simulink library "mbd_s32k1xx_ec_toolbox"  (Simulink 9.0)
settings: Solver=FixedStepDiscrete  StartTime=0.0  StopTime=10.0  FixedStep=0.1  RelTol=1e-3  EnableMultiTasking=on
InitFcn:
  | mbd_s32k_consistency_checks(bdroot(gcs));
(part 1 of 8)
settings Model: Creator=r61406  LastModifiedBy=nxf35172

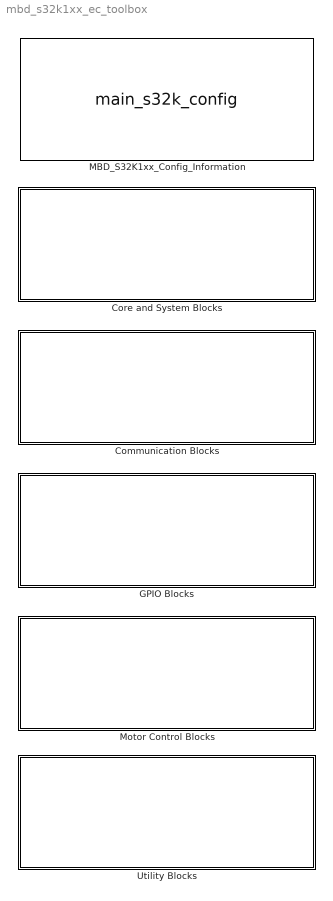
== system mbd_s32k1xx_ec_toolbox ==
  Communication Blocks : Subsystem
  Core and System Blocks : Subsystem
  GPIO Blocks : Subsystem
  MBD_S32K1xx_Config_Information : S-Function  LoadFcn=|  InitFcn=|  FunctionName=main_s32k_config  SFunctionDeploymentMode=off  EnableBusSupport=off  mask(MBDTBX_EC_S32K){mbdt_ver=0, disp_str=|, config_params=[], mcu_target_name=S32K148, mcu_target_package=100-LQFP, mcu_target_sram_size=192KB, mcu_system_clock_freq=80, mcu_xtal_freq=External 8, mcu_steptick_timer=LPIT Channel 0, mcu_steptick_prio=15, ds_import_enable=on, target_compiler=GCC, target_memory=FLASH, gcc_target_compile_opts=-mthumb -mfloat-abi=hard -mfpu=fpv4-sp-d16 -O1 -g -gstrict-dwarf, gcc_target_assemble_opts=-mthumb -mfloat-abi=hard -mfpu=fpv4-sp-d16 -g, gcc_target_link_opts=-mthumb -mfloat-abi=hard -mfpu=fpv4-sp-d16, gcc_target_lib_opts=, gcc_target_default_lcf=on, gcc_target_user_lcf=S32K148_192_flash.ld, ghs_target_compile_opts=-cpu=cortexm4f -thumb -fpu=vfpv4_d16 -fsingle -Ogeneral -Wundef -Wimplicit-int -Wshadow -Wtrigraphs --no_commons --gnu_asm -gnu99 -gdwarf-2 -G, ghs_target_assemble_opts=-cpu=cortexm4f -fpu=vfpv4_d16, ghs_target_link_opts=-cpu=cortexm4f -thumb -fpu=vfpv4_d16, ghs_target_lib_opts=, ghs_target_default_lcf=on, ghs_target_user_lcf=S32K148_192_flash.ld, iar_target_compile_opts=--cpu=Cortex-M4F --thumb --fpu=VFPv4_sp -Ol -e --debug --dlib_config normal, iar_target_assemble_opts=--cpu Cortex-M4F --thumb --fpu VFPv4_sp, iar_target_link_opts=--no_exceptions --vfe --inline, iar_target_lib_opts=, iar_target_default_lcf=on, iar_target_user_lcf=S32K148_192_flash.icf, pil_download_enable=off, rbl_download_enable=off, rbl_start_delay=5000, rbl_download_interface=OpenSDA, rbl_restart_request=off, rbl_com_port=Custom, rbl_com_port_custom=COM1, pil_download_rate=57600, pil_opensda_drive=Custom, pil_opensda_drive_custom=D, pil_uart_instance=1, pil_uart_rx=PTC6: [LPUART1_RX | Receive], pil_uart_tx=PTC7: [LPUART1_TX | Transmit], FTM_PWM_PcrCheckEnDis=on, FTM_Input_Edge_Inputs_PcrCheckEnDis=on, FTM_Dual_Edge_Inputs_PcrCheckEnDis=on, FTM_Quadrature_Inputs_PcrCheckEnDis=on, FTM_Hall_Sensor_Inputs_PcrCheckEnDis=on, LPTMR_PcrCheckEnDis=on, PIT_PcrCheckEnDis=on, RTC_PcrCheckEnDis=on, FlexCAN_PcrCheckEnDis=on, LIN_PcrCheckEnDis=on, FlexIO_PcrCheckEnDis=on, LPI2C_PcrCheckEnDis=on, LPSPI_PcrCheckEnDis=on, LPUART_PcrCheckEnDis=on, CMP_PcrCheckEnDis=on, GPIO_OutputPcrCheckEnDis=on, GPIO_InputPcrCheckEnDis=on, SBC_PcrCheckEnDis=on, AMMCLIB_PcrCheckEnDis=on, FM_PcrCheckEnDis=on, Profile_PcrCheckEnDis=on, ConfigParams_PcrCheckEnDis=on, ModelRef_PcrCheckEnDis=on, PDB0_PcrCheckEnDis=on, CSEc_PcrCheckEnDis=on, eDMA_PcrCheckEnDis=on, ADC_PcrCheckEnDis=on, WDOG_PcrCheckEnDis=on}
      LoadFcn=|
      | mbd_s32k_set_cur_model(bdroot(gcs));
      | mbd_s32k_block_load(bdroot(gcs));
      InitFcn=|
      | mbd_s32k_set_cur_model(bdroot(gcs)); 
      | mbd_s32k_update_model('init');       
      | mbd_s32k_check('MBDTBX_EC_S32K14');
      mask disp_str=|
      | Target : S32K144-64KB_SRAM
      | Package : 100-pin
      | System clock : 80 MHz
      | XTAL clock : External 8 MHz
      | Compiler : IAR
      | Target Type : FLASH
      | Download Code after build : off
      | Step Tick Interrupt Priority : 15
      mask prompts: mbdt_ver "MBDT Version"; disp_str "display_string"; mcu_target_name "Family"; mcu_target_package "Package"; mcu_target_sram_size "SRAM"; mcu_system_clock_freq "Clock Frequency MHz"; mcu_xtal_freq "XTAL Frequency MHz"; mcu_steptick_timer "Timer"; mcu_steptick_prio "Priority"; ds_import_enable "Generate S32 Design Studio ProjectInfo.xml file"; target_compiler "Compiler"; target_memory "Target Memory Model"; gcc_target_compile_opts "Compile Options"; gcc_target_assemble_opts "Assemble Options"; gcc_target_link_opts "Link Options"; gcc_target_lib_opts "Library Options"; gcc_target_default_lcf "Default Target Memory Definitions"; gcc_target_user_lcf "User Defined Target Memory Definitions"; ghs_target_compile_opts "Compile Options"; ghs_target_assemble_opts "Assemble Options"; ghs_target_link_opts "Link Options"; ghs_target_lib_opts "Library Options"; ghs_target_default_lcf "Default Target Memory Definitions"; ghs_target_user_lcf "User Defined Target Memory Definitions"; iar_target_compile_opts "Compile Options"; iar_target_assemble_opts "Assemble Options"; iar_target_link_opts "Link Options"; iar_target_lib_opts "Library Options"; iar_target_default_lcf "Default Target Memory Definitions"; iar_target_user_lcf "User Defined Target Memory Definitions"; pil_download_enable "Processor-in-the-Loop (PIL) Mode Download"; rbl_download_enable "Download Code after Build"; rbl_start_delay "Delay before start of application (ms)"; rbl_download_interface "Download Interface"; rbl_restart_request "Boot Assist Module (BAM) Restart Request"; rbl_com_port "COM Port"; rbl_com_port_custom "Custom COM Port"; pil_download_rate "Baud Rate"; pil_opensda_drive "OpenSDA Drive Name"; pil_opensda_drive_custom "Custom OpenSDA Drive Name"; pil_uart_instance "LPUART"; pil_uart_rx "RX pin"; pil_uart_tx "TX pin"; FTM_PWM_PcrCheckEnDis "FTM PWM Config"; FTM_Input_Edge_Inputs_PcrCheckEnDis "FTM Input Edge Inputs"; FTM_Dual_Edge_Inputs_PcrCheckEnDis "FTM Dual Edge Inputs"; FTM_Quadrature_Inputs_PcrCheckEnDis "FTM Quadrature Inputs"; FTM_Hall_Sensor_Inputs_PcrCheckEnDis "FTM Hall Sensor Inputs"; LPTMR_PcrCheckEnDis "LPTMR"; PIT_PcrCheckEnDis "PIT"; RTC_PcrCheckEnDis "RTC"; FlexCAN_PcrCheckEnDis "FlexCAN"; LIN_PcrCheckEnDis "LIN"; FlexIO_PcrCheckEnDis "FlexIO"; LPI2C_PcrCheckEnDis "LPI2C"; LPSPI_PcrCheckEnDis "LPSPI"; LPUART_PcrCheckEnDis "LPUART"; CMP_PcrCheckEnDis "CMP"; GPIO_OutputPcrCheckEnDis "GPIO Output"; GPIO_InputPcrCheckEnDis "GPIO Input"; SBC_PcrCheckEnDis "SBC"; AMMCLIB_PcrCheckEnDis "AMMCLIB"; FM_PcrCheckEnDis "FreeMaster"; Profile_PcrCheckEnDis "Profile"; ConfigParams_PcrCheckEnDis "Config Params"; ModelRef_PcrCheckEnDis "Model Reference"; PDB0_PcrCheckEnDis "PDB"; CSEc_PcrCheckEnDis "CSEc"; eDMA_PcrCheckEnDis "eDMA"; ADC_PcrCheckEnDis "ADC"; WDOG_PcrCheckEnDis "WDOG"
      mask help: Model-Based Design Toolbox Config block for S32K1xx family of processors.
      mask init:
      | mbd_s32k_config_com_ports_cbk('populate_drop_down');
      | maskStr = mbd_s32k_mb_display_string();
      settings: NameChangeFcn=mbd_s32k_model_close;
      settings: CopyFcn=|
      | mbd_s32k_set_cur_model(bdroot(gcs));
      | mbd_s32k_check('MBDTBX_EC_S32K');
      | mbd_s32k_update_model('copy');
      settings: ModelCloseFcn=|
      | mbd_s32k_set_cur_model(bdroot(gcs));
      | mbd_s32k_model_close;
      settings: CloseFcn=|
      | mbd_s32k_set_cur_model(bdroot(gcs));
      | mbd_s32k_check('MBDTBX_EC_S32K');
      | mbd_s32k_update_model('copy');
      mask Help: web(fullfile(mbd_s32k_block_help, 'main_config', 'main_config.html'));
      mask TypeOptions mcu_target_name: S32K116 | S32K118 | S32K142 | S32K144 | S32K146 | S32K148
      mask Callback mcu_target_name:
      | mbd_s32k_config_target_cbk('mcu_target_name');
      | mbd_s32k_config_target_cbk('mcu_target_compiler');
      | mbd_s32k_config_target_cbk('mcu_target_memory');
      mask TypeOptions mcu_target_package: 100-LQFP | 144-LQFP | 176-LQFP | 100-BGA
      mask Callback mcu_target_package: mbd_s32k_config_target_cbk('mcu_target_package')
      mask TypeOptions mcu_target_sram_size: 192KB | 256KB
      mask Callback mcu_target_sram_size: mbd_s32k_config_target_cbk('mcu_target_sram_size')
      mask TypeOptions mcu_system_clock_freq: 80 | 112
      mask TypeOptions mcu_xtal_freq: External 8 | External 40
      mask TypeOptions mcu_steptick_timer: LPIT Channel 0 | Suppress
      mask TypeOptions mcu_steptick_prio: 15 | 14 | 13 | 12 | 11 | 10 | 9 | 8 | 7 | 6 | 5 | 4 | 3 | 2 | 1 | 0
      mask TypeOptions target_compiler: GCC | IAR | GreenHills Multi
      mask Callback target_compiler: mbd_s32k_config_compiler_cbk('target_compiler')
      mask TypeOptions target_memory: FLASH | SRAM
      mask Callback target_memory: mbd_s32k_config_memory_cbk('target_memory')
      mask Callback gcc_target_default_lcf: mbd_s32k_config_lcf_cbk('gcc_target_default_lcf')
      mask TypeOptions gcc_target_user_lcf: S32K148_192_flash.ld | S32K148_192_flash_bam.ld
      mask TypeOptions ghs_target_user_lcf: S32K148_192_flash.ld | S32K148_192_flash_bam.ld
      mask Callback iar_target_default_lcf: mbd_s32k_config_lcf_cbk('iar_target_default_lcf')
      mask TypeOptions iar_target_user_lcf: S32K148_192_flash.icf | S32K148_192_flash_bam.icf
      mask Callback pil_download_enable: mbd_s32k_config_pil_cbk('pil_download_enable')
      mask Callback rbl_download_enable: mbd_s32k_config_pil_cbk('rbl_download_enable');
      mask TypeOptions rbl_download_interface: Serial | OpenSDA
      mask Callback rbl_download_interface: mbd_s32k_config_pil_cbk('rbl_download_interface')
      mask TypeOptions rbl_com_port: COM1 | COM17 | Custom
      mask Callback rbl_com_port: mbd_s32k_config_com_ports_cbk('populate_drop_down')
      mask TypeOptions pil_download_rate: 9600 | 14400 | 19200 | 38400 | 56000 | 57600 | 115200
      mask TypeOptions pil_opensda_drive: D: S32K116EVB | Custom
      mask Callback pil_opensda_drive:
      | mbd_s32k_config_vol_disks_cbk('populate_drop_down');
      | mbd_s32k_config_vol_disks_cbk('enable_custom');
      mask TypeOptions pil_uart_instance: 0 | 1 | 2
      mask Callback pil_uart_instance: mbd_s32k_config_pil_cbk('pil_uart_instance');
      mask TypeOptions pil_uart_rx: PTA2: [LPUART0_RX | Receive] | PTB0: [LPUART0_RX | Receive] | PTC2: [LPUART0_RX | Receive] | PTC6: [LPUART1_RX | Receive] | PTC8: [LPUART1_RX | Receive] | PTA2: [LPUART0_RX | Receive] | PTB0: [LPUART0_RX | Receive] | PTC2: [LPUART0_RX | Receive] | PTC6: [LPUART1_RX | Receive] | PTC8: [LPUART1_RX | Receive] | PTA2: [LPUART0_RX | Receive] | PTB0: [LPUART0_RX | Receive] | PTC2: [LPUART0_RX | Receive] | PTC6: [LPUART1_RX | Receive] | PTC8: [LPUART1_RX | Receive] | PTA2: [LPUART0_RX | Receive] | PTB0: [LPUART0_RX | Receive] | PTC2: [LPUART0_RX | Receive] | PTC6: [LPUART1_RX | Receive] | PTC8: [LPUART1_RX | Receive] | PTA8: [LPUART2_RX | Receive] | PTD6: [LPUART2_RX | Receive] | PTD17: [LPUART2_RX | Receive] | PTA2: [LPUART0_RX | Receive] | PTB0: [LPUART0_RX | Receive] | PTC2: [LPUART0_RX | Receive] | PTC6: [LPUART1_RX | Receive] | PTC8: [LPUART1_RX | Receive] | PTA8: [LPUART2_RX | Receive] | PTD6: [LPUART2_RX | Receive] | PTD17: [LPUART2_RX | Receive] | PTA2: [LPUART0_RX | Receive] | PTB0: [LPUART0_RX | Receive] | PTC2: [LPUART0_RX | Receive] | PTC6: [LPUART1_RX | Receive] | PTC8: [LPUART1_RX | Receive] | PTA8: [LPUART2_RX | Receive] | PTD6: [LPUART2_RX | Receive] | PTD17: [LPUART2_RX | Receive]
      mask TypeOptions pil_uart_tx: PTA3: [LPUART0_TX | Transmit] | PTB1: [LPUART0_TX | Transmit] | PTC3: [LPUART0_TX | Transmit] | PTC7: [LPUART1_TX | Transmit] | PTC9: [LPUART1_TX | Transmit] | PTA3: [LPUART0_TX | Transmit] | PTB1: [LPUART0_TX | Transmit] | PTC3: [LPUART0_TX | Transmit] | PTC7: [LPUART1_TX | Transmit] | PTC9: [LPUART1_TX | Transmit] | PTA3: [LPUART0_TX | Transmit] | PTB1: [LPUART0_TX | Transmit] | PTC3: [LPUART0_TX | Transmit] | PTC7: [LPUART1_TX | Transmit] | PTC9: [LPUART1_TX | Transmit] | PTA3: [LPUART0_TX | Transmit] | PTB1: [LPUART0_TX | Transmit] | PTC3: [LPUART0_TX | Transmit] | PTC7: [LPUART1_TX | Transmit] | PTC9: [LPUART1_TX | Transmit] | PTA9: [LPUART2_TX | Transmit] | PTD7: [LPUART2_TX | Transmit] | PTE12: [LPUART2_TX | Transmit] | PTA3: [LPUART0_TX | Transmit] | PTB1: [LPUART0_TX | Transmit] | PTC3: [LPUART0_TX | Transmit] | PTC7: [LPUART1_TX | Transmit] | PTC9: [LPUART1_TX | Transmit] | PTA9: [LPUART2_TX | Transmit] | PTD7: [LPUART2_TX | Transmit] | PTE12: [LPUART2_TX | Transmit] | PTA3: [LPUART0_TX | Transmit] | PTB1: [LPUART0_TX | Transmit] | PTC3: [LPUART0_TX | Transmit] | PTC7: [LPUART1_TX | Transmit] | PTC9: [LPUART1_TX | Transmit] | PTA9: [LPUART2_TX | Transmit] | PTD7: [LPUART2_TX | Transmit] | PTE12: [LPUART2_TX | Transmit]
      mask DialogControl Container14 Prompt: Target MCU
      mask DialogControl Container15 Prompt: Clock
      mask DialogControl Container16 Prompt: Step Tick
      mask DialogControl propagate_configuration Prompt: Propagate configuration
      mask DialogControl propagate_configuration Tooltip: Press this button to propagate the settings to all referenced models.
      mask DialogControl propagate_configuration Callback: mbd_s32k_config_propagate_cbk(gcb);
      mask DialogControl rbl_com_button Prompt: Refresh
      mask DialogControl rbl_com_button Callback: mbd_s32k_config_com_ports_cbk('populate_drop_down')
      mask DialogControl pil_opensda_refresh Prompt: Refresh
      mask DialogControl pil_opensda_refresh Callback: mbd_s32k_config_vol_disks_cbk('populate_drop_down')
      mask DialogControl Container17 Prompt: Consistency checks
      mask Display:
      | image('nxp_logo.png', 'top-right');
      | disp(maskStr);
  Motor Control Blocks : Subsystem
  Utility Blocks : Subsystem

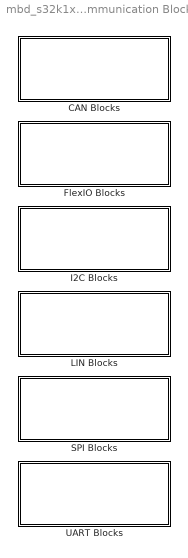
== system mbd_s32k1xx_ec_toolbox/Communication Blocks ==
  CAN Blocks : Subsystem
  "FlexIO Blocks " : Subsystem
  I2C Blocks : Subsystem
  LIN Blocks : Subsystem
  SPI Blocks : Subsystem
  UART Blocks : Subsystem

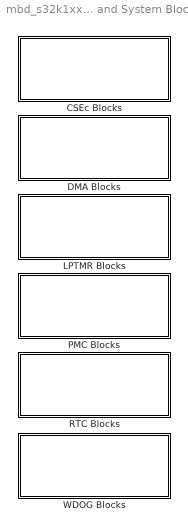
== system mbd_s32k1xx_ec_toolbox/Core and System Blocks ==
  CSEc Blocks : Subsystem
  DMA Blocks : Subsystem
  LPTMR Blocks : Subsystem
  PMC Blocks : Subsystem
  RTC Blocks : Subsystem
  WDOG Blocks : Subsystem

== system mbd_s32k1xx_ec_toolbox/GPIO Blocks ==
  Digital_Input : S-Function  FunctionName=gpio_s32k_input  SFunctionDeploymentMode=off  EnableBusSupport=off  mask(gpio_s32k_input){gpio_pin=PTA0: [PTA0 | Port A I/O], pull_resistor=None, passive_filter=off}
      mask prompts: gpio_pin "Input Pin"; pull_resistor "Pull Resistor Select"; passive_filter "Passive Filter Enable"
      mask help: Select a General Purpose Input Pin as a Source.
      mask init:
      | mbd_s32k_gpi_init;
      settings: NameChangeFcn=mbd_s32k_name_check (gcb);
      mask Help: web(fullfile(mbd_s32k_block_help, 'gpio', 'gpio_input.html'));
      mask TypeOptions gpio_pin: PTA0: [PTA0 | Port A I/O] | PTA1: [PTA1 | Port A I/O] | PTA2: [PTA2 | Port A I/O] | PTA3: [PTA3 | Port A I/O] | PTA4: [PTA4 | Port A I/O] | PTA5: [PTA5 | Port A I/O] | PTA6: [PTA6 | Port A I/O] | PTA7: [PTA7 | Port A I/O] | PTA8: [PTA8 | Port A I/O] | PTA9: [PTA9 | Port A I/O] | PTA10: [PTA10 | Port A I/O] | PTA11: [PTA11 | Port A I/O] | PTA12: [PTA12 | Port A I/O] | PTA13: [PTA13 | Port A I/O] | PTA14: [PTA14 | Port A I/O] | PTA15: [PTA15 | Port A I/O] | PTA16: [PTA16 | Port A I/O] | PTA17: [PTA17 | Port A I/O] | PTA18: [PTA18 | Port A I/O] | PTA19: [PTA19 | Port A I/O] | PTA20: [PTA20 | Port A I/O] | PTA21: [PTA21 | Port A I/O] | PTA22: [PTA22 | Port A I/O] | PTA23: [PTA23 | Port A I/O] | PTA24: [PTA24 | Port A I/O] | PTA25: [PTA25 | Port A I/O] | PTA26: [PTA26 | Port A I/O] | PTA27: [PTA27 | Port A I/O] | PTA28: [PTA28 | Port A I/O] | PTA29: [PTA29 | Port A I/O] | PTA30: [PTA30 | Port A I/O] | PTA31: [PTA31 | Port A I/O] | PTB0: [PTB0 | Port B I/O] | PTB1: [PTB1 | Port B I/O] | PTB2: [PTB2 | Port B I/O] | PTB3: [PTB3 | Port B I/O] | PTB4: [PTB4 | Port B I/O] | PTB5: [PTB5 | Port B I/O] | PTB6: [PTB6 | Port B I/O] | PTB7: [PTB7 | Port B I/O] | PTB8: [PTB8 | Port B I/O] | PTB9: [PTB9 | Port B I/O] | PTB10: [PTB10 | Port B I/O] | PTB11: [PTB11 | Port B I/O] | PTB12: [PTB12 | Port B I/O] | PTB13: [PTB13 | Port B I/O] | PTB14: [PTB14 | Port B I/O] | PTB15: [PTB15 | Port B I/O] | PTB16: [PTB16 | Port B I/O] | PTB17: [PTB17 | Port B I/O] | PTB18: [PTB18 | Port B I/O] | PTB19: [PTB19 | Port B I/O] | PTB20: [PTB20 | Port B I/O] | PTB21: [PTB21 | Port B I/O] | PTB22: [PTB22 | Port B I/O] | PTB23: [PTB23 | Port B I/O] | PTB24: [PTB24 | Port B I/O] | PTB25: [PTB25 | Port B I/O] | PTB26: [PTB26 | Port B I/O] | PTB27: [PTB27 | Port B I/O] | PTB28: [PTB28 | Port B I/O] | PTB29: [PTB29 | Port B I/O] | PTB30: [PTB30 | Port B I/O] | PTB31: [PTB31 | Port B I/O] | PTC0: [PTC0 | Port C I/O] | PTC1: [PTC1 | Port C I/O] | PTC2: [PTC2 | Port C I/O] | PTC3: [PTC3 | Port C I/O] | PTC4: [PTC4 | Port C I/O] | PTC5: [PTC5 | Port C I/O] | PTC6: [PTC6 | Port C I/O] | PTC7: [PTC7 | Port C I/O] | PTC8: [PTC8 | Port C I/O] | PTC9: [PTC9 | Port C I/O] | PTC10: [PTC10 | Port C I/O] | PTC11: [PTC11 | Port C I/O] | PTC12: [PTC12 | Port C I/O] | PTC13: [PTC13 | Port C I/O] | PTC14: [PTC14 | Port C I/O] | PTC15: [PTC15 | Port C I/O] | PTC16: [PTC16 | Port C I/O] | PTC17: [PTC17 | Port C I/O] | PTC18: [PTC18 | Port C I/O] | PTC19: [PTC19 | Port C I/O] | PTC20: [PTC20 | Port C I/O] | PTC21: [PTC21 | Port C I/O] | PTC22: [PTC22 | Port C I/O] | PTC23: [PTC23 | Port C I/O] | PTC24: [PTC24 | Port C I/O] | PTC25: [PTC25 | Port C I/O] | PTC26: [PTC26 | Port C I/O] | PTC27: [PTC27 | Port C I/O] | PTC28: [PTC28 | Port C I/O] | PTC29: [PTC29 | Port C I/O] | PTC30: [PTC30 | Port C I/O] | PTC31: [PTC31 | Port C I/O] | PTD0: [PTD0 | Port D I/O] | PTD1: [PTD1 | Port D I/O] | PTD2: [PTD2 | Port D I/O] | PTD3: [PTD3 | Port D I/O] | PTD4: [PTD4 | Port D I/O] | PTD5: [PTD5 | Port D I/O] | PTD6: [PTD6 | Port D I/O] | PTD7: [PTD7 | Port D I/O] | PTD8: [PTD8 | Port D I/O] | PTD9: [PTD9 | Port D I/O] | PTD10: [PTD10 | Port D I/O] | PTD11: [PTD11 | Port D I/O] | PTD12: [PTD12 | Port D I/O] | PTD13: [PTD13 | Port D I/O] | PTD14: [PTD14 | Port D I/O] | PTD15: [PTD15 | Port D I/O] | PTD16: [PTD16 | Port D I/O] | PTD17: [PTD17 | Port D I/O] | PTD18: [PTD18 | Port D I/O] | PTD19: [PTD19 | Port D I/O] | PTD20: [PTD20 | Port D I/O] | PTD21: [PTD21 | Port D I/O] | PTD22: [PTD22 | Port D I/O] | PTD23: [PTD23 | Port D I/O] | PTD24: [PTD24 | Port D I/O] | PTD25: [PTD25 | Port D I/O] | PTD26: [PTD26 | Port D I/O] | PTD27: [PTD27 | Port D I/O] | PTD28: [PTD28 | Port D I/O] | PTD29: [PTD29 | Port D I/O] | PTD30: [PTD30 | Port D I/O] | PTD31: [PTD31 | Port D I/O] | PTE0: [PTE0 | Port E I/O] | PTE1: [PTE1 | Port E I/O] | PTE2: [PTE2 | Port E I/O] | PTE3: [PTE3 | Port E I/O] | PTE4: [PTE4 | Port E I/O] | PTE5: [PTE5 | Port E I/O] | PTE6: [PTE6 | Port E I/O] | PTE7: [PTE7 | Port E I/O] | PTE8: [PTE8 | Port E I/O] | PTE9: [PTE9 | Port E I/O] | PTE10: [PTE10 | Port E I/O] | PTE11: [PTE11 | Port E I/O] | PTE12: [PTE12 | Port E I/O] | PTE13: [PTE13 | Port E I/O] | PTE14: [PTE14 | Port E I/O] | PTE15: [PTE15 | Port E I/O] | PTE16: [PTE16 | Port E I/O] | PTE17: [PTE17 | Port E I/O] | PTE18: [PTE18 | Port E I/O] | PTE19: [PTE19 | Port E I/O] | PTE20: [PTE20 | Port E I/O] | PTE21: [PTE21 | Port E I/O] | PTE22: [PTE22 | Port E I/O] | PTE23: [PTE23 | Port E I/O] | PTE24: [PTE24 | Port E I/O] | PTE25: [PTE25 | Port E I/O] | PTE26: [PTE26 | Port E I/O] | PTE27: [PTE27 | Port E I/O]
      mask Callback gpio_pin: mbd_s32k_display_pin_info('gpio', gcb, 'gpio_pin')
      mask TypeOptions pull_resistor: None | Pulldown | Pullup
      mask Display:
      | image('nxp_logo.png', 'top-right');
      | port_label('output',1,'input');
      | disp(maskStr);
  Digital_Input_ISR : S-Function  FunctionName=gpi_s32k_isr  SFunctionDeploymentMode=off  EnableBusSupport=off  mask(gpi_s32k_isr){gpio_pin=PTA0: [PTA0 | Port A I/O], irqc=when logic 0, prio=15}
      mask prompts: gpio_pin "Input Pin"; irqc "Interrupt Configuration"; prio "ISR Priority"
      mask help: Configure a General Purpose Input Pin to generate an ISR.
      mask init:
      | mbd_s32k_gpi_isr_init;
      settings: NameChangeFcn=mbd_s32k_name_check (gcb);
      mask Help: web(fullfile(mbd_s32k_block_help, 'gpio', 'gpi_isr.html'));
      mask TypeOptions gpio_pin: PTA0: [PTA0 | Port A I/O] | PTA1: [PTA1 | Port A I/O] | PTA2: [PTA2 | Port A I/O] | PTA3: [PTA3 | Port A I/O] | PTA4: [PTA4 | Port A I/O] | PTA5: [PTA5 | Port A I/O] | PTA6: [PTA6 | Port A I/O] | PTA7: [PTA7 | Port A I/O] | PTA8: [PTA8 | Port A I/O] | PTA9: [PTA9 | Port A I/O] | PTA10: [PTA10 | Port A I/O] | PTA11: [PTA11 | Port A I/O] | PTA12: [PTA12 | Port A I/O] | PTA13: [PTA13 | Port A I/O] | PTA14: [PTA14 | Port A I/O] | PTA15: [PTA15 | Port A I/O] | PTA16: [PTA16 | Port A I/O] | PTA17: [PTA17 | Port A I/O] | PTA18: [PTA18 | Port A I/O] | PTA19: [PTA19 | Port A I/O] | PTA20: [PTA20 | Port A I/O] | PTA21: [PTA21 | Port A I/O] | PTA22: [PTA22 | Port A I/O] | PTA23: [PTA23 | Port A I/O] | PTA24: [PTA24 | Port A I/O] | PTA25: [PTA25 | Port A I/O] | PTA26: [PTA26 | Port A I/O] | PTA27: [PTA27 | Port A I/O] | PTA28: [PTA28 | Port A I/O] | PTA29: [PTA29 | Port A I/O] | PTA30: [PTA30 | Port A I/O] | PTA31: [PTA31 | Port A I/O] | PTB0: [PTB0 | Port B I/O] | PTB1: [PTB1 | Port B I/O] | PTB2: [PTB2 | Port B I/O] | PTB3: [PTB3 | Port B I/O] | PTB4: [PTB4 | Port B I/O] | PTB5: [PTB5 | Port B I/O] | PTB6: [PTB6 | Port B I/O] | PTB7: [PTB7 | Port B I/O] | PTB8: [PTB8 | Port B I/O] | PTB9: [PTB9 | Port B I/O] | PTB10: [PTB10 | Port B I/O] | PTB11: [PTB11 | Port B I/O] | PTB12: [PTB12 | Port B I/O] | PTB13: [PTB13 | Port B I/O] | PTB14: [PTB14 | Port B I/O] | PTB15: [PTB15 | Port B I/O] | PTB16: [PTB16 | Port B I/O] | PTB17: [PTB17 | Port B I/O] | PTB18: [PTB18 | Port B I/O] | PTB19: [PTB19 | Port B I/O] | PTB20: [PTB20 | Port B I/O] | PTB21: [PTB21 | Port B I/O] | PTB22: [PTB22 | Port B I/O] | PTB23: [PTB23 | Port B I/O] | PTB24: [PTB24 | Port B I/O] | PTB25: [PTB25 | Port B I/O] | PTB26: [PTB26 | Port B I/O] | PTB27: [PTB27 | Port B I/O] | PTB28: [PTB28 | Port B I/O] | PTB29: [PTB29 | Port B I/O] | PTB30: [PTB30 | Port B I/O] | PTB31: [PTB31 | Port B I/O] | PTC0: [PTC0 | Port C I/O] | PTC1: [PTC1 | Port C I/O] | PTC2: [PTC2 | Port C I/O] | PTC3: [PTC3 | Port C I/O] | PTC4: [PTC4 | Port C I/O] | PTC5: [PTC5 | Port C I/O] | PTC6: [PTC6 | Port C I/O] | PTC7: [PTC7 | Port C I/O] | PTC8: [PTC8 | Port C I/O] | PTC9: [PTC9 | Port C I/O] | PTC10: [PTC10 | Port C I/O] | PTC11: [PTC11 | Port C I/O] | PTC12: [PTC12 | Port C I/O] | PTC13: [PTC13 | Port C I/O] | PTC14: [PTC14 | Port C I/O] | PTC15: [PTC15 | Port C I/O] | PTC16: [PTC16 | Port C I/O] | PTC17: [PTC17 | Port C I/O] | PTC18: [PTC18 | Port C I/O] | PTC19: [PTC19 | Port C I/O] | PTC20: [PTC20 | Port C I/O] | PTC21: [PTC21 | Port C I/O] | PTC22: [PTC22 | Port C I/O] | PTC23: [PTC23 | Port C I/O] | PTC24: [PTC24 | Port C I/O] | PTC25: [PTC25 | Port C I/O] | PTC26: [PTC26 | Port C I/O] | PTC27: [PTC27 | Port C I/O] | PTC28: [PTC28 | Port C I/O] | PTC29: [PTC29 | Port C I/O] | PTC30: [PTC30 | Port C I/O] | PTC31: [PTC31 | Port C I/O] | PTD0: [PTD0 | Port D I/O] | PTD1: [PTD1 | Port D I/O] | PTD2: [PTD2 | Port D I/O] | PTD3: [PTD3 | Port D I/O] | PTD4: [PTD4 | Port D I/O] | PTD5: [PTD5 | Port D I/O] | PTD6: [PTD6 | Port D I/O] | PTD7: [PTD7 | Port D I/O] | PTD8: [PTD8 | Port D I/O] | PTD9: [PTD9 | Port D I/O] | PTD10: [PTD10 | Port D I/O] | PTD11: [PTD11 | Port D I/O] | PTD12: [PTD12 | Port D I/O] | PTD13: [PTD13 | Port D I/O] | PTD14: [PTD14 | Port D I/O] | PTD15: [PTD15 | Port D I/O] | PTD16: [PTD16 | Port D I/O] | PTD17: [PTD17 | Port D I/O] | PTD18: [PTD18 | Port D I/O] | PTD19: [PTD19 | Port D I/O] | PTD20: [PTD20 | Port D I/O] | PTD21: [PTD21 | Port D I/O] | PTD22: [PTD22 | Port D I/O] | PTD23: [PTD23 | Port D I/O] | PTD24: [PTD24 | Port D I/O] | PTD25: [PTD25 | Port D I/O] | PTD26: [PTD26 | Port D I/O] | PTD27: [PTD27 | Port D I/O] | PTD28: [PTD28 | Port D I/O] | PTD29: [PTD29 | Port D I/O] | PTD30: [PTD30 | Port D I/O] | PTD31: [PTD31 | Port D I/O] | PTE0: [PTE0 | Port E I/O] | PTE1: [PTE1 | Port E I/O] | PTE2: [PTE2 | Port E I/O] | PTE3: [PTE3 | Port E I/O] | PTE4: [PTE4 | Port E I/O] | PTE5: [PTE5 | Port E I/O] | PTE6: [PTE6 | Port E I/O] | PTE7: [PTE7 | Port E I/O] | PTE8: [PTE8 | Port E I/O] | PTE9: [PTE9 | Port E I/O] | PTE10: [PTE10 | Port E I/O] | PTE11: [PTE11 | Port E I/O] | PTE12: [PTE12 | Port E I/O] | PTE13: [PTE13 | Port E I/O] | PTE14: [PTE14 | Port E I/O] | PTE15: [PTE15 | Port E I/O] | PTE16: [PTE16 | Port E I/O] | PTE17: [PTE17 | Port E I/O] | PTE18: [PTE18 | Port E I/O] | PTE19: [PTE19 | Port E I/O] | PTE20: [PTE20 | Port E I/O] | PTE21: [PTE21 | Port E I/O] | PTE22: [PTE22 | Port E I/O] | PTE23: [PTE23 | Port E I/O] | PTE24: [PTE24 | Port E I/O] | PTE25: [PTE25 | Port E I/O] | PTE26: [PTE26 | Port E I/O] | PTE27: [PTE27 | Port E I/O]
      mask Callback gpio_pin: mbd_s32k_display_pin_info('gpio', gcb, 'gpio_pin')
      mask TypeOptions irqc: when logic 0 | on rising-edge | on falling-edge | on either-edge | when logic 1
      mask TypeOptions prio: 0 | 1 | 2 | 3 | 4 | 5 | 6 | 7 | 8 | 9 | 10 | 11 | 12 | 13 | 14 | 15
      mask Callback prio: mbd_s32k_isr_priority_cbk(gcb, 'prio')
      mask Display:
      | image('nxp_logo.png', 'top-right');
      | port_label('output',1,'function');
      | disp(maskStr);
  Digital_Input_ISR_Enable_Disable : S-Function  FunctionName=gpi_s32k_isr_control  SFunctionDeploymentMode=off  EnableBusSupport=off  mask(gpi_s32k_isr_control){gpio_pin=PTA0: [PTA0 | Port A I/O], irqc=request disabled}
      mask prompts: gpio_pin "Input Pin"; irqc "Interrupt Configuration"
      mask help: This block enables or disables the interrupt for GPI ISR block.
      mask init:
      | mbd_s32k_gpi_isr_control_init;
      settings: NameChangeFcn=mbd_s32k_name_check(gcb);
      mask Help: web(fullfile(mbd_s32k_block_help, 'gpio', 'gpi_isr_control.html'));
      mask TypeOptions gpio_pin: PTA0: [PTA0 | Port A I/O] | PTA1: [PTA1 | Port A I/O] | PTA2: [PTA2 | Port A I/O] | PTA3: [PTA3 | Port A I/O] | PTA4: [PTA4 | Port A I/O] | PTA5: [PTA5 | Port A I/O] | PTA6: [PTA6 | Port A I/O] | PTA7: [PTA7 | Port A I/O] | PTA8: [PTA8 | Port A I/O] | PTA9: [PTA9 | Port A I/O] | PTA10: [PTA10 | Port A I/O] | PTA11: [PTA11 | Port A I/O] | PTA12: [PTA12 | Port A I/O] | PTA13: [PTA13 | Port A I/O] | PTA14: [PTA14 | Port A I/O] | PTA15: [PTA15 | Port A I/O] | PTA16: [PTA16 | Port A I/O] | PTA17: [PTA17 | Port A I/O] | PTA18: [PTA18 | Port A I/O] | PTA19: [PTA19 | Port A I/O] | PTA20: [PTA20 | Port A I/O] | PTA21: [PTA21 | Port A I/O] | PTA22: [PTA22 | Port A I/O] | PTA23: [PTA23 | Port A I/O] | PTA24: [PTA24 | Port A I/O] | PTA25: [PTA25 | Port A I/O] | PTA26: [PTA26 | Port A I/O] | PTA27: [PTA27 | Port A I/O] | PTA28: [PTA28 | Port A I/O] | PTA29: [PTA29 | Port A I/O] | PTA30: [PTA30 | Port A I/O] | PTA31: [PTA31 | Port A I/O] | PTB0: [PTB0 | Port B I/O] | PTB1: [PTB1 | Port B I/O] | PTB2: [PTB2 | Port B I/O] | PTB3: [PTB3 | Port B I/O] | PTB4: [PTB4 | Port B I/O] | PTB5: [PTB5 | Port B I/O] | PTB6: [PTB6 | Port B I/O] | PTB7: [PTB7 | Port B I/O] | PTB8: [PTB8 | Port B I/O] | PTB9: [PTB9 | Port B I/O] | PTB10: [PTB10 | Port B I/O] | PTB11: [PTB11 | Port B I/O] | PTB12: [PTB12 | Port B I/O] | PTB13: [PTB13 | Port B I/O] | PTB14: [PTB14 | Port B I/O] | PTB15: [PTB15 | Port B I/O] | PTB16: [PTB16 | Port B I/O] | PTB17: [PTB17 | Port B I/O] | PTB18: [PTB18 | Port B I/O] | PTB19: [PTB19 | Port B I/O] | PTB20: [PTB20 | Port B I/O] | PTB21: [PTB21 | Port B I/O] | PTB22: [PTB22 | Port B I/O] | PTB23: [PTB23 | Port B I/O] | PTB24: [PTB24 | Port B I/O] | PTB25: [PTB25 | Port B I/O] | PTB26: [PTB26 | Port B I/O] | PTB27: [PTB27 | Port B I/O] | PTB28: [PTB28 | Port B I/O] | PTB29: [PTB29 | Port B I/O] | PTB30: [PTB30 | Port B I/O] | PTB31: [PTB31 | Port B I/O] | PTC0: [PTC0 | Port C I/O] | PTC1: [PTC1 | Port C I/O] | PTC2: [PTC2 | Port C I/O] | PTC3: [PTC3 | Port C I/O] | PTC4: [PTC4 | Port C I/O] | PTC5: [PTC5 | Port C I/O] | PTC6: [PTC6 | Port C I/O] | PTC7: [PTC7 | Port C I/O] | PTC8: [PTC8 | Port C I/O] | PTC9: [PTC9 | Port C I/O] | PTC10: [PTC10 | Port C I/O] | PTC11: [PTC11 | Port C I/O] | PTC12: [PTC12 | Port C I/O] | PTC13: [PTC13 | Port C I/O] | PTC14: [PTC14 | Port C I/O] | PTC15: [PTC15 | Port C I/O] | PTC16: [PTC16 | Port C I/O] | PTC17: [PTC17 | Port C I/O] | PTC18: [PTC18 | Port C I/O] | PTC19: [PTC19 | Port C I/O] | PTC20: [PTC20 | Port C I/O] | PTC21: [PTC21 | Port C I/O] | PTC22: [PTC22 | Port C I/O] | PTC23: [PTC23 | Port C I/O] | PTC24: [PTC24 | Port C I/O] | PTC25: [PTC25 | Port C I/O] | PTC26: [PTC26 | Port C I/O] | PTC27: [PTC27 | Port C I/O] | PTC28: [PTC28 | Port C I/O] | PTC29: [PTC29 | Port C I/O] | PTC30: [PTC30 | Port C I/O] | PTC31: [PTC31 | Port C I/O] | PTD0: [PTD0 | Port D I/O] | PTD1: [PTD1 | Port D I/O] | PTD2: [PTD2 | Port D I/O] | PTD3: [PTD3 | Port D I/O] | PTD4: [PTD4 | Port D I/O] | PTD5: [PTD5 | Port D I/O] | PTD6: [PTD6 | Port D I/O] | PTD7: [PTD7 | Port D I/O] | PTD8: [PTD8 | Port D I/O] | PTD9: [PTD9 | Port D I/O] | PTD10: [PTD10 | Port D I/O] | PTD11: [PTD11 | Port D I/O] | PTD12: [PTD12 | Port D I/O] | PTD13: [PTD13 | Port D I/O] | PTD14: [PTD14 | Port D I/O] | PTD15: [PTD15 | Port D I/O] | PTD16: [PTD16 | Port D I/O] | PTD17: [PTD17 | Port D I/O] | PTD18: [PTD18 | Port D I/O] | PTD19: [PTD19 | Port D I/O] | PTD20: [PTD20 | Port D I/O] | PTD21: [PTD21 | Port D I/O] | PTD22: [PTD22 | Port D I/O] | PTD23: [PTD23 | Port D I/O] | PTD24: [PTD24 | Port D I/O] | PTD25: [PTD25 | Port D I/O] | PTD26: [PTD26 | Port D I/O] | PTD27: [PTD27 | Port D I/O] | PTD28: [PTD28 | Port D I/O] | PTD29: [PTD29 | Port D I/O] | PTD30: [PTD30 | Port D I/O] | PTD31: [PTD31 | Port D I/O] | PTE0: [PTE0 | Port E I/O] | PTE1: [PTE1 | Port E I/O] | PTE2: [PTE2 | Port E I/O] | PTE3: [PTE3 | Port E I/O] | PTE4: [PTE4 | Port E I/O] | PTE5: [PTE5 | Port E I/O] | PTE6: [PTE6 | Port E I/O] | PTE7: [PTE7 | Port E I/O] | PTE8: [PTE8 | Port E I/O] | PTE9: [PTE9 | Port E I/O] | PTE10: [PTE10 | Port E I/O] | PTE11: [PTE11 | Port E I/O] | PTE12: [PTE12 | Port E I/O] | PTE13: [PTE13 | Port E I/O] | PTE14: [PTE14 | Port E I/O] | PTE15: [PTE15 | Port E I/O] | PTE16: [PTE16 | Port E I/O] | PTE17: [PTE17 | Port E I/O] | PTE18: [PTE18 | Port E I/O] | PTE19: [PTE19 | Port E I/O] | PTE20: [PTE20 | Port E I/O] | PTE21: [PTE21 | Port E I/O] | PTE22: [PTE22 | Port E I/O] | PTE23: [PTE23 | Port E I/O] | PTE24: [PTE24 | Port E I/O] | PTE25: [PTE25 | Port E I/O] | PTE26: [PTE26 | Port E I/O] | PTE27: [PTE27 | Port E I/O]
      mask Callback gpio_pin: mbd_s32k_display_pin_info('gpio', gcb, 'gpio_pin')
      mask TypeOptions irqc: request disabled | when logic 0 | on rising-edge | on falling-edge | on either-edge | when logic 1
      mask Display:
      | image('nxp_logo.png', 'top-right');
      | disp(maskStr);
  Digital_Output : S-Function  FunctionName=gpio_s32k_output  SFunctionDeploymentMode=off  EnableBusSupport=off  mask(gpio_s32k_output){gpio_pin=PTA0: [PTA0 | Port A I/O], init_val=Low, drive_strength=Low}
      mask prompts: gpio_pin "Output Pin"; init_val "Initial value"; drive_strength "Drive Strength"
      mask help: Select a General Purpose Output Pin as a Sink.
      mask init:
      | mbd_s32k_gpo_init;
      settings: NameChangeFcn=mbd_s32k_name_check (gcb);
      mask Help: web(fullfile(mbd_s32k_block_help, 'gpio', 'gpio_output.html'));
      mask TypeOptions gpio_pin: PTA0: [PTA0 | Port A I/O] | PTA1: [PTA1 | Port A I/O] | PTA2: [PTA2 | Port A I/O] | PTA3: [PTA3 | Port A I/O] | PTA4: [PTA4 | Port A I/O] | PTA5: [PTA5 | Port A I/O] | PTA6: [PTA6 | Port A I/O] | PTA7: [PTA7 | Port A I/O] | PTA8: [PTA8 | Port A I/O] | PTA9: [PTA9 | Port A I/O] | PTA10: [PTA10 | Port A I/O] | PTA11: [PTA11 | Port A I/O] | PTA12: [PTA12 | Port A I/O] | PTA13: [PTA13 | Port A I/O] | PTA14: [PTA14 | Port A I/O] | PTA15: [PTA15 | Port A I/O] | PTA16: [PTA16 | Port A I/O] | PTA17: [PTA17 | Port A I/O] | PTA18: [PTA18 | Port A I/O] | PTA19: [PTA19 | Port A I/O] | PTA20: [PTA20 | Port A I/O] | PTA21: [PTA21 | Port A I/O] | PTA22: [PTA22 | Port A I/O] | PTA23: [PTA23 | Port A I/O] | PTA24: [PTA24 | Port A I/O] | PTA25: [PTA25 | Port A I/O] | PTA26: [PTA26 | Port A I/O] | PTA27: [PTA27 | Port A I/O] | PTA28: [PTA28 | Port A I/O] | PTA29: [PTA29 | Port A I/O] | PTA30: [PTA30 | Port A I/O] | PTA31: [PTA31 | Port A I/O] | PTB0: [PTB0 | Port B I/O] | PTB1: [PTB1 | Port B I/O] | PTB2: [PTB2 | Port B I/O] | PTB3: [PTB3 | Port B I/O] | PTB4: [PTB4 | Port B I/O] | PTB5: [PTB5 | Port B I/O] | PTB6: [PTB6 | Port B I/O] | PTB7: [PTB7 | Port B I/O] | PTB8: [PTB8 | Port B I/O] | PTB9: [PTB9 | Port B I/O] | PTB10: [PTB10 | Port B I/O] | PTB11: [PTB11 | Port B I/O] | PTB12: [PTB12 | Port B I/O] | PTB13: [PTB13 | Port B I/O] | PTB14: [PTB14 | Port B I/O] | PTB15: [PTB15 | Port B I/O] | PTB16: [PTB16 | Port B I/O] | PTB17: [PTB17 | Port B I/O] | PTB18: [PTB18 | Port B I/O] | PTB19: [PTB19 | Port B I/O] | PTB20: [PTB20 | Port B I/O] | PTB21: [PTB21 | Port B I/O] | PTB22: [PTB22 | Port B I/O] | PTB23: [PTB23 | Port B I/O] | PTB24: [PTB24 | Port B I/O] | PTB25: [PTB25 | Port B I/O] | PTB26: [PTB26 | Port B I/O] | PTB27: [PTB27 | Port B I/O] | PTB28: [PTB28 | Port B I/O] | PTB29: [PTB29 | Port B I/O] | PTB30: [PTB30 | Port B I/O] | PTB31: [PTB31 | Port B I/O] | PTC0: [PTC0 | Port C I/O] | PTC1: [PTC1 | Port C I/O] | PTC2: [PTC2 | Port C I/O] | PTC3: [PTC3 | Port C I/O] | PTC4: [PTC4 | Port C I/O] | PTC5: [PTC5 | Port C I/O] | PTC6: [PTC6 | Port C I/O] | PTC7: [PTC7 | Port C I/O] | PTC8: [PTC8 | Port C I/O] | PTC9: [PTC9 | Port C I/O] | PTC10: [PTC10 | Port C I/O] | PTC11: [PTC11 | Port C I/O] | PTC12: [PTC12 | Port C I/O] | PTC13: [PTC13 | Port C I/O] | PTC14: [PTC14 | Port C I/O] | PTC15: [PTC15 | Port C I/O] | PTC16: [PTC16 | Port C I/O] | PTC17: [PTC17 | Port C I/O] | PTC18: [PTC18 | Port C I/O] | PTC19: [PTC19 | Port C I/O] | PTC20: [PTC20 | Port C I/O] | PTC21: [PTC21 | Port C I/O] | PTC22: [PTC22 | Port C I/O] | PTC23: [PTC23 | Port C I/O] | PTC24: [PTC24 | Port C I/O] | PTC25: [PTC25 | Port C I/O] | PTC26: [PTC26 | Port C I/O] | PTC27: [PTC27 | Port C I/O] | PTC28: [PTC28 | Port C I/O] | PTC29: [PTC29 | Port C I/O] | PTC30: [PTC30 | Port C I/O] | PTC31: [PTC31 | Port C I/O] | PTD0: [PTD0 | Port D I/O] | PTD1: [PTD1 | Port D I/O] | PTD2: [PTD2 | Port D I/O] | PTD3: [PTD3 | Port D I/O] | PTD4: [PTD4 | Port D I/O] | PTD5: [PTD5 | Port D I/O] | PTD6: [PTD6 | Port D I/O] | PTD7: [PTD7 | Port D I/O] | PTD8: [PTD8 | Port D I/O] | PTD9: [PTD9 | Port D I/O] | PTD10: [PTD10 | Port D I/O] | PTD11: [PTD11 | Port D I/O] | PTD12: [PTD12 | Port D I/O] | PTD13: [PTD13 | Port D I/O] | PTD14: [PTD14 | Port D I/O] | PTD15: [PTD15 | Port D I/O] | PTD16: [PTD16 | Port D I/O] | PTD17: [PTD17 | Port D I/O] | PTD18: [PTD18 | Port D I/O] | PTD19: [PTD19 | Port D I/O] | PTD20: [PTD20 | Port D I/O] | PTD21: [PTD21 | Port D I/O] | PTD22: [PTD22 | Port D I/O] | PTD23: [PTD23 | Port D I/O] | PTD24: [PTD24 | Port D I/O] | PTD25: [PTD25 | Port D I/O] | PTD26: [PTD26 | Port D I/O] | PTD27: [PTD27 | Port D I/O] | PTD28: [PTD28 | Port D I/O] | PTD29: [PTD29 | Port D I/O] | PTD30: [PTD30 | Port D I/O] | PTD31: [PTD31 | Port D I/O] | PTE0: [PTE0 | Port E I/O] | PTE1: [PTE1 | Port E I/O] | PTE2: [PTE2 | Port E I/O] | PTE3: [PTE3 | Port E I/O] | PTE4: [PTE4 | Port E I/O] | PTE5: [PTE5 | Port E I/O] | PTE6: [PTE6 | Port E I/O] | PTE7: [PTE7 | Port E I/O] | PTE8: [PTE8 | Port E I/O] | PTE9: [PTE9 | Port E I/O] | PTE10: [PTE10 | Port E I/O] | PTE11: [PTE11 | Port E I/O] | PTE12: [PTE12 | Port E I/O] | PTE13: [PTE13 | Port E I/O] | PTE14: [PTE14 | Port E I/O] | PTE15: [PTE15 | Port E I/O] | PTE16: [PTE16 | Port E I/O] | PTE17: [PTE17 | Port E I/O] | PTE18: [PTE18 | Port E I/O] | PTE19: [PTE19 | Port E I/O] | PTE20: [PTE20 | Port E I/O] | PTE21: [PTE21 | Port E I/O] | PTE22: [PTE22 | Port E I/O] | PTE23: [PTE23 | Port E I/O] | PTE24: [PTE24 | Port E I/O] | PTE25: [PTE25 | Port E I/O] | PTE26: [PTE26 | Port E I/O] | PTE27: [PTE27 | Port E I/O]
      mask Callback gpio_pin: mbd_s32k_display_pin_info('gpio', gcb, 'gpio_pin')
      mask TypeOptions init_val: Low | High
      mask TypeOptions drive_strength: Low | High
      mask Display:
      | image('nxp_logo.png', 'top-right');
      | disp(st);
      | port_label('input',1,'output');

== system mbd_s32k1xx_ec_toolbox/Motor Control Blocks ==
  ADC Blocks : Subsystem
  CMP Blocks : Subsystem
  FTM Blocks : Subsystem
  PDB Blocks : Subsystem
